simulink model "ControlRM20"  (R2020a)
settings: Solver=VariableStepAuto  StartTime=0.0  StopTime=inf  RelTol=1e-3
undefined symbols (not defined in the file): Standard_Devices, UDP_Protocol, v, w
libraries: sldrtlib x2
settings Model: Creator=alrer  LastModifiedBy=alrer

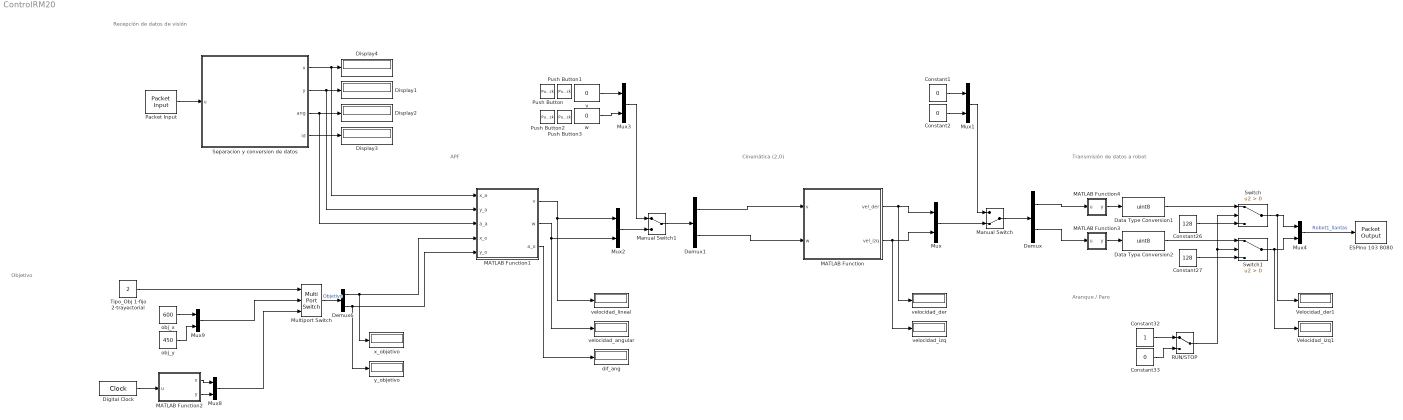
== system ControlRM20 ==
  note: Cinemática (2,0)
  note: Transmisión de datos a robot
  note: Aranque / Paro
  note: APF
  note: Objetivo
  note: Recepción de datos de visión
  Constant1 : Constant  Value=0
  Constant2 : Constant  Value=0
  Constant26 : Constant  Value=128
  Constant27 : Constant  Value=128
  Constant32 : Constant
  Constant33 : Constant  Value=0
  Data Type Conversion1 : DataTypeConversion  OutMin=0  OutMax=255  OutDataTypeStr=uint8
  Data Type Conversion2 : DataTypeConversion  OutMin=0  OutMax=255  OutDataTypeStr=uint8
  Demux : Demux  Outputs=2
  Demux1 : Demux  Outputs=2
  Demux6 : Demux  Outputs=2
  Digital Clock : DigitalClock  SampleTime=-1
  Display{1..4} (4 alike) : Display
  ESPino 103 8080 : sldrtlib/Packet Output  SampleTime=0.01  MaxMissedTicks=inf  ShowMissedTicks=off  YieldWhenWaiting=off  DrvName=Standard_Devices/UDP_Protocol  DrvAddress=12001  DrvOptions=[0 8080 49 57 50 46 49 54 56 46 49 51 55 46 49 55 49 0 0 0 0 0 0 0 0 0 0 0 0 0 0 0 0 0 0 0 0 0 0 0 0 0 0 0 0 0 0 0 0 0 0 0 0 0 0 0 0 0 0 0 0 0 0 0 0 0 0 0 0 0 0 0 0 0 0 0 0 0 0 0 0 0 0 0 0 0 0 0 0 0 0 0 0 0 0 0 0 0 0 0 0 0 0 0 0 0 0 0 0 0 0 0 0 0 0 0 0 0 0 0 0 0 0 0 0 0 0 0 0 0 0 0 0 0 0 0 0 0 0 0 0 0 0 0 0 0 0 0 0 0 0 0 0 0 0 0 0 0 0 0 0 0 0 0 0 0 0 0 0 0 0 0 0 0 0 0 0 0 0 0 0 0 0 0 0 0 0 0 0 0 0 0 0 0 0 0 0 0 0 0 0 0 0 0 0 0 0 0 0 0 0 0 0 0 0 0 0 0 0 0 0 0 0 0 0 0 0 0 0 0 0 0 0 0 0 0 0 0 0 0 0 0 0 0 0 0 0 0 0 0 0 0 0 0 0 0]  PacketSize=2  DataTypes='2*uint8'  ShowReady=off  ShowError=off  PacketID=1  ByteOrder=1  InitialValue=[]  FinalValue=[]
      settings: AttributesFormatString=UDP Protocol [12001]
  MATLAB Function : MATLAB Function  TreatAsAtomicUnit=on
  MATLAB Function1 : MATLAB Function  TreatAsAtomicUnit=on
  MATLAB Function2 : MATLAB Function  TreatAsAtomicUnit=on
  MATLAB Function3 : MATLAB Function  TreatAsAtomicUnit=on
  MATLAB Function4 : MATLAB Function  TreatAsAtomicUnit=on
  Manual Switch : ManualSwitch  CurrentSetting=0
  Manual Switch1 : ManualSwitch
  Multiport Switch : MultiPortSwitch  Inputs=2  DiagnosticForDefault=Warning
  Mux{,1..4,8..9} (7 alike) : Mux  Inputs=2
  Packet Input : sldrtlib/Packet Input  SampleTime=0.001  MaxMissedTicks=inf  ShowMissedTicks=off  YieldWhenWaiting=off  DrvName=Standard_Devices/UDP_Protocol  DrvAddress=58624  DrvOptions=[0 58624 49 50 55 46 48 46 48 46 49 0 0 0 0 0 0 0 0 0 0 0 0 0 0 0 0 0 0 0 0 0 0 0 0 0 0 0 0 0 0 0 0 0 0 0 0 0 0 0 0 0 0 0 0 0 0 0 0 0 0 0 0 0 0 0 0 0 0 0 0 0 0 0 0 0 0 0 0 0 0 0 0 0 0 0 0 0 0 0 0 0 0 0 0 0 0 0 0 0 0 0 0 0 0 0 0 0 0 0 0 0 0 0 0 0 0 0 0 0 0 0 0 0 0 0 0 0 0 0 0 0 0 0 0 0 0 0 0 0 0 0 0 0 0 0 0 0 0 0 0 0 0 0 0 0 0 0 0 0 0 0 0 0 0 0 0 0 0 0 0 0 0 0 0 0 0 0 0 0 0 0 0 0 0 0 0 0 0 0 0 0 0 0 0 0 0 0 0 0 0 0 0 0 0 0 0 0 0 0 0 0 0 0 0 0 0 0 0 0 0 0 0 0 0 0 0 0 0 0 0 0 0 0 0 0 0 0 0 0 0 0 0 0 0 0 0 0 0 0 0 0 0 0 0 0]  PacketSize=34  DataTypes='34*int8'  ShowReady=off  ShowError=off  PacketID=1  ByteOrder=1  ShowTimestamp=off
      settings: AttributesFormatString=UDP Protocol [58624]
  Push Button : PushButtonBlock  ButtonText=v-  OnValue=-500
  Push Button1 : PushButtonBlock  ButtonText=v+  OnValue=500
  Push Button2 : PushButtonBlock  ButtonText=w-  OnValue=-5
  Push Button3 : PushButtonBlock  ButtonText=w+  OnValue=5
  RUN/STOP : ManualSwitch
  Separacion y conversion de datos : MATLAB Function  TreatAsAtomicUnit=on
  Switch : Switch  Criteria=u2 > Threshold
  Switch1 : Switch  Criteria=u2 > Threshold
  Tipo_Obj 1-fijo 2-trayectorial : Constant  Value=2
  "Velocidad_der1 " : Display
  Velocidad_izq1 : Display
  dif_ang : Display
  obj_x : Constant  Value=600
  obj_y : Constant  Value=450
  v : Constant  Value=0
  velocidad_angular : Display
  velocidad_der : Display
  velocidad_izq : Display
  velocidad_lineal : Display
  w : Constant  Value=0
  x_objetivo : Display
  y_objetivo : Display
  wires:
  Packet Input/1 -> Separacion y conversion de datos/1(u)
  Separacion y conversion de datos/1(x) -> MATLAB Function1/1(x_a), Display4/1
  Separacion y conversion de datos/2(y) -> Display1/1, MATLAB Function1/2(y_a)
  Separacion y conversion de datos/3(ang) -> Display2/1, MATLAB Function1/3(a_a)
  Separacion y conversion de datos/4(id) -> Display3/1
  Switch1/1 -> Velocidad_izq1/1, Mux4/2
  Constant26/1 -> Switch/3
  Switch/1 -> "Velocidad_der1 "/1, Mux4/1
  Constant27/1 -> Switch1/3
  Mux4/1 -> ESPino 103 8080/1  "Robot1_llantas"
  Constant32/1 -> RUN/STOP/1
  Constant33/1 -> RUN/STOP/2
  RUN/STOP/1 -> Switch/2, Switch1/2
  MATLAB Function1/1(v) -> velocidad_lineal/1, Mux2/1
  MATLAB Function1/2(w) -> velocidad_angular/1, Mux2/2
  Multiport Switch/1 -> Demux6/1  "Objetivo"
  Digital Clock/1 -> MATLAB Function2/1(u)
  MATLAB Function2/1(x) -> Mux8/1
  Mux9/1 -> Multiport Switch/2
  obj_x/1 -> Mux9/1
  MATLAB Function2/2(y) -> Mux8/2
  Mux8/1 -> Multiport Switch/3
  Tipo_Obj 1-fijo 2-trayectorial/1 -> Multiport Switch/1
  obj_y/1 -> Mux9/2
  Demux6/1 -> x_objetivo/1, MATLAB Function1/4(x_o)
  Demux6/2 -> y_objetivo/1, MATLAB Function1/5(y_o)
  MATLAB Function/1(vel_der) -> velocidad_der/1, Mux/1
  MATLAB Function/2(vel_izq) -> velocidad_izq/1, Mux/2
  Mux/1 -> Manual Switch/2
  Manual Switch/1 -> Demux/1
  Demux/2 -> MATLAB Function3/1(u)
  Demux/1 -> MATLAB Function4/1(u)
  Constant2/1 -> Mux1/2
  Constant1/1 -> Mux1/1
  Mux1/1 -> Manual Switch/1
  Manual Switch1/1 -> Demux1/1
  Mux2/1 -> Manual Switch1/2
  Demux1/1 -> MATLAB Function/1(v)
  Demux1/2 -> MATLAB Function/2(w)
  w/1 -> Mux3/2
  Mux3/1 -> Manual Switch1/1
  MATLAB Function3/1(y) -> Data Type Conversion2/1
  v/1 -> Mux3/1
  MATLAB Function4/1(y) -> Data Type Conversion1/1
  Data Type Conversion1/1 -> Switch/1
  Data Type Conversion2/1 -> Switch1/1
  MATLAB Function1/3(a_o) -> dif_ang/1

== matlab function ControlRM20/MATLAB Function ==
  data: v input; vel_der output; w input; vel_izq output
function [vel_der, vel_izq] = fcn(v, w)

    % Parametros Robot
    r = 60;               % Radio de las llantas [mm]
    b = 85;               % Distancia del eje de desplazamiento del robot al centro de las llantas [mm]
    d = 60;               % Distancia del eje de las llantas al punto de control en la dirección de desplazamiento [mm]

    velMax = 100;         % Velocidad máxima de giro de las llantas
    
    % Cálculo de las velocidades de giro de las llantas
    vLlantaDer = (v + b*w)/r; % Velocidad de giro de la llanta derecha   Signo - por ajuste de los motores
    vLlantaIzq = (v - b*w)/r; % Velocidad de giro de la llanta izquierda
      
    % Límite de la velocidad máxima
    if (vLlantaDer > velMax)
        vLlantaDer = velMax;
    elseif (vLlantaDer < -velMax)
        vLlantaDer = -velMax;
    end
      
    if (vLlantaIzq > velMax)
        vLlantaIzq = velMax;
    elseif (vLlantaIzq < -velMax)
        vLlantaIzq = -velMax;
    end
    
    vel_der = vLlantaDer;
    vel_izq = vLlantaIzq;
    
%********************* Ajuste para tarjetas md25   ************************

    %vel_der = 128 + vLlantaDer;
    %vel_izq = 128 + vLlantaIzq;
    
end

== matlab function ControlRM20/Separacion y conversion de datos ==
  data: u input; x output; y output; ang output; id output
function [x, y, ang, id] = fcn(u)
    aux=0;
    e=zeros(17);

    for i=1:1:17
        if u(i)==77 % Identificador de inicio de cadena "M"
            aux=i;
        end
    end
    
    r=17;
    for j=1:1:r
        e(j)=u(aux+j);
    end

    id = e(16)-48;
    x=(e(2)-48)*1000+(e(3)-48)*100+(e(4)-48)*10+(e(5)-48);
    y=(e(7)-48)*1000+(e(8)-48)*100+(e(9)-48)*10+(e(10)-48);
    ang=(e(13)-48)*100 + (e(14)-48)*10 + (e(15)-48);

    if(e(1)==45)
           x = -x;
    end

    if(e(6)==45)
           y = -y;
    end
end

== matlab function ControlRM20/MATLAB Function1 ==
  data: x_a input; v output; y_a input; a_a input; x_o input; y_o input; w output; a_o output
function [v, w, a_o] = fcn(x_a, y_a, a_a, x_o, y_o)

    kv = 1.5;        % Constante de proporcionalidad de velocidad lineal
    kw = 0.1;          % Constante de proporcionalidad de velocidad angular
    rp = 30;         % Radio de protección del robot (se considera que ya llegó al objetivo) [mm]
    ap = 15;         % Ángulo de protección [°]
    

    d_obj=sqrt((x_o-x_a)^2+(y_o-y_a)^2);  %Calcula la distancia del agente al objetivo
    v = kv * d_obj;            %Velocidad hacia el objetivo es proporcional a la distancia al mismo
      
    a_o = atan2(y_o-y_a, x_o-x_a)*180/pi;    %Cálculo del ángulo con respecto al eje x del agente al objetivo
    da_obj = a_o - (a_a + 90);         %Diferencia entre ángulo del agente y ángulo al objetivo
    
    if (da_obj > 180)
        da_obj = da_obj - 360;
    end
      
    if (da_obj < -180)
        da_obj = da_obj + 360;
    end
    
    w = kw * da_obj;            %Velocidad angular es proporcional a diferencia de ángulo
    
    if (d_obj < rp)
        v = 0;
    end
    if (abs(da_obj) < ap)
        w = 0;
    end

end

== matlab function ControlRM20/MATLAB Function3 ==
  data: u input; y output
function y = fcn(u)

y = 128-u;

== matlab function ControlRM20/MATLAB Function4 ==
  data: u input; y output
function y = fcn(u)

y = 128 + u;

== matlab function ControlRM20/MATLAB Function2 ==
  data: x output; u input; y output
function [x,y] = trayectoria(u)
    x = 300*cos(u/10)+600;
    y = 300*sin(u/10)+450;

end
